simulink model "Test"  (R2016a)
settings: Solver=VariableStepAuto  StartTime=0.0  StopTime=100.0  MinStep=0.01  RelTol=1e-3
values from neighbouring files (symbols this model uses):
  b = 0.01    [fa.m]    (also in finalprogram.m; results.m)
  j = 0.1    [fa.m]    (also in finalprogram.m; results.m)
  ld = 0.0009    [fa.m]    (also in finalprogram.m; results.m)
  lmbdm = 0.14    [fa.m]    (also in finalprogram.m; results.m)
  lq = 0.0009    [fa.m]    (also in finalprogram.m; results.m)
  MA = zeros(3,3)    [programlinear.m]
  MB = zeros(3,2)    [programlinear.m]
  MC = eye(3)    [results.m]
  MD = zeros(3,2)    [results.m]
  n = 18    [fa.m]    (also in finalprogram.m; results.m)
  rs = 1.3    [fa.m]    (also in finalprogram.m; results.m)
  u1 = x0(3)    [finalprogram.m]    (also in programlinear.m = result(3); results.m = result(3))
  U1O = u1    [results.m]
  u2 = x0(4)    [finalprogram.m]    (also in programlinear.m = result(4); results.m = result(4))
  U2O = u2    [results.m]
  x1 = x0(1)    [finalprogram.m]    (also in programlinear.m = result(1); results.m = result(1))
  x2 = x0(2)    [finalprogram.m]    (also in programlinear.m = result(2); results.m = result(2))
  x3 = 20    [results.m]
settings Model: Creator=manoe  LastModifiedBy=manoe

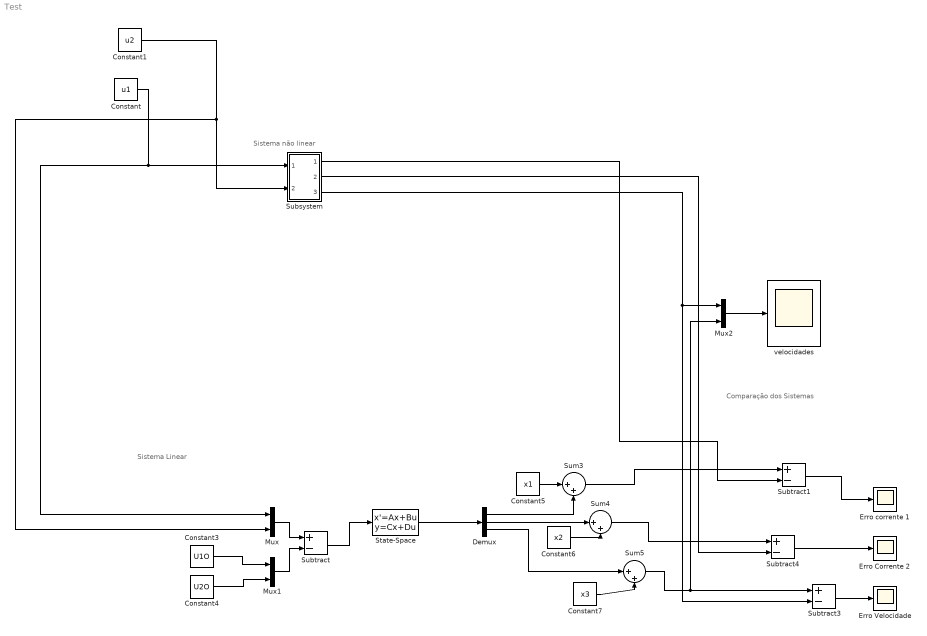
== system Test ==
  note: Comparação dos Sistemas
  note: Sistema Linear
  note: Sistema não linear
  Constant : Constant  Value=u1
  Constant1 : Constant  Value=u2
  Constant3 : Constant  Value=U1O
  Constant4 : Constant  Value=U2O
  Constant5 : Constant  Value=x1
  Constant6 : Constant  Value=x2
  Constant7 : Constant  Value=x3
  Demux : Demux  Outputs=3
  Erro Corrente 2 : Scope
  Erro Velocidade : Scope
  Erro corrente 1 : Scope
  Mux : Mux  Inputs=2
  Mux1 : Mux  Inputs=2
  Mux2 : Mux  Inputs=2
  State-Space : StateSpace  A=MA  B=MB  C=MC  D=MD  X0=0
  Subsystem : Subsystem
  Subtract{,1,3..4} (4 alike) : Sum  Inputs=+-
  Sum3 : Sum  Inputs=|++
  Sum4 : Sum  Inputs=|++
  Sum5 : Sum  Inputs=|++
  "velocidades " : Scope
  wires:
  Constant/1 -> Mux/1, Subsystem/1(In1)
  Constant1/1 -> Subsystem/2(In2), Mux/2
  Mux/1 -> Subtract/1
  Mux1/1 -> Subtract/2
  Constant3/1 -> Mux1/1
  Constant4/1 -> Mux1/2
  Subtract/1 -> State-Space/1
  State-Space/1 -> Demux/1
  Demux/1 -> Sum3/2
  Constant5/1 -> Sum3/1
  Demux/2 -> Sum4/1
  Constant6/1 -> Sum4/2
  Demux/3 -> Sum5/1
  Constant7/1 -> Sum5/2
  Sum3/1 -> Subtract1/1
  Sum4/1 -> Subtract4/1
  Sum5/1 -> Subtract3/1, Mux2/2
  Subtract1/1 -> Erro corrente 1/1
  Subtract4/1 -> Erro Corrente 2/1
  Subtract3/1 -> Erro Velocidade/1
  Subsystem/1(Out1) -> Subtract1/2
  Subsystem/2(Out2) -> Subtract4/2
  Subsystem/3(Out3) -> Subtract3/2, Mux2/1
  Mux2/1 -> "velocidades "/1

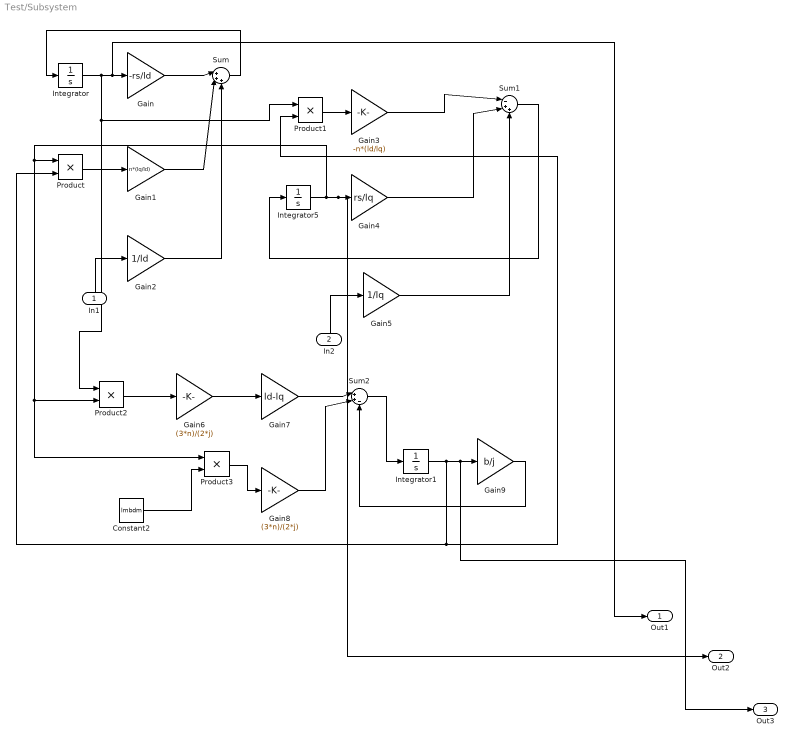
== system Test/Subsystem ==
  In1 : Inport
  In2 : Inport  Port=2
  Constant2 : Constant  Value=lmbdm
  Gain : Gain  Gain=-rs/ld
  Gain1 : Gain  Gain=n*(lq/ld)
  Gain2 : Gain  Gain=1/ld
  Gain3 : Gain  Gain=-n*(ld/lq)
  Gain4 : Gain  Gain=rs/lq
  Gain5 : Gain  Gain=1/lq
  Gain6 : Gain  Gain=(3*n)/(2*j)
  Gain7 : Gain  Gain=ld-lq
  Gain8 : Gain  Gain=(3*n)/(2*j)
  Gain9 : Gain  Gain=b/j
  Integrator : Integrator  InitialCondition=x1
  Integrator1 : Integrator  InitialCondition=x3
  Integrator5 : Integrator  InitialCondition=x2
  Product{,1..3} (4 alike) : Product
  Sum : Sum  Inputs=|+++
  Sum1 : Sum  Inputs=|-++
  Sum2 : Sum  Inputs=|++-
  Out1 : Outport
  Out2 : Outport  Port=2
  Out3 : Outport  Port=3
  wires:
  Integrator/1 -> Product2/1, Product1/1, Out1/1, Gain/1
  Gain2/1 -> Sum/3
  In1/1 -> Gain2/1
  In2/1 -> Gain5/1
  Gain/1 -> Sum/1
  Sum/1 -> Integrator/1
  Product/1 -> Gain1/1
  Gain1/1 -> Sum/2
  Product1/1 -> Gain3/1
  Gain3/1 -> Sum1/1
  Integrator5/1 -> Product/1, Product2/2, Product3/1, Out2/1, Gain4/1
  Gain8/1 -> Sum2/2
  Constant2/1 -> Product3/2
  Sum1/1 -> Integrator5/1
  Gain4/1 -> Sum1/2
  Product3/1 -> Gain8/1
  Gain5/1 -> Sum1/3
  Integrator1/1 -> Product1/2, Product/2, Out3/1, Gain9/1
  Gain7/1 -> Sum2/1
  Gain6/1 -> Gain7/1
  Sum2/1 -> Integrator1/1
  Product2/1 -> Gain6/1
  Gain9/1 -> Sum2/3
